simulink model "PID"  (R2024a)
settings: Solver=VariableStepAuto  StartTime=0.0  StopTime=11  RelTol=1e-3
settings Model: Creator=thunguyen  LastModifiedBy=thunguyen

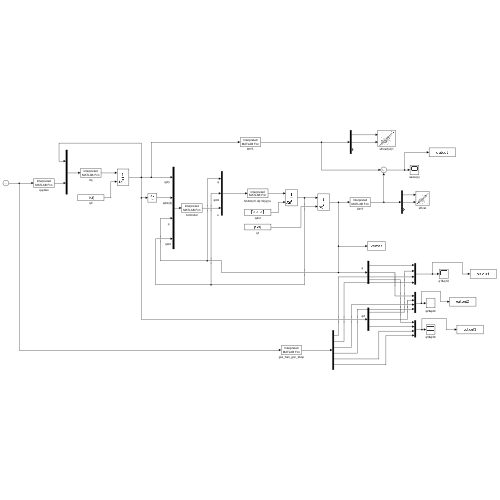
[thumbnail: Simulink's stored preview of the top-level diagram]
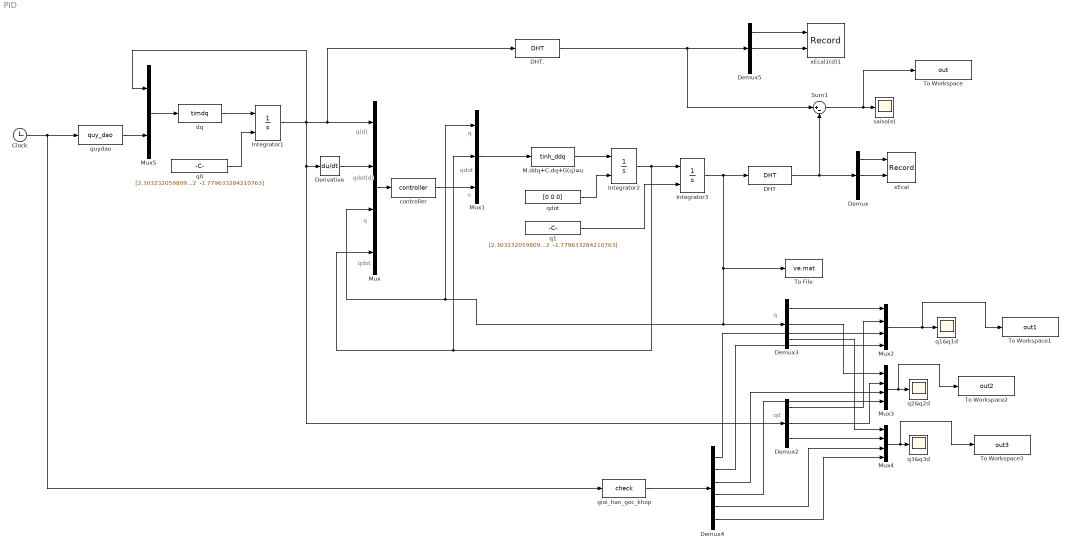
== system PID ==
  note: qd
  note: q
  note: u
  note: qdot
  note: qdot(d)
  note: q
  note: q
  note: q(d)
  note: qdot
  Clock : Clock
      settings: Decimation=2
  DHT : MATLABFcn  MATLABFcn=DHT  OutputDimensions=3  Output1D=off
  DHT. : MATLABFcn  MATLABFcn=DHT  OutputDimensions=3  Output1D=off
  Demux{,2..3,5} (4 alike) : Demux  Outputs=3
  Demux4 : Demux  Outputs=6
  Derivative : Derivative
  Integrator1 : Integrator  InitialConditionSource=external  InitialCondition=1
  Integrator2 : Integrator  InitialConditionSource=external  InitialCondition=1
  Integrator3 : Integrator  InitialConditionSource=external  InitialCondition=1
  M.ddq+C.dq+G(q)=u : MATLABFcn  MATLABFcn=tinh_ddq  OutputDimensions=3  Output1D=off
  Mux{,2..4} (4 alike) : Mux
  Mux1 : Mux  Inputs=3
  Mux5 : Mux  Inputs=2
  Sum1 : Sum  Inputs=|+-
  To File : ToFile  Filename=ve.mat
  To Workspace : ToWorkspace  VariableName=out  SaveFormat=Timeseries  SampleTime=-1
  To Workspace1 : ToWorkspace  VariableName=out1  SaveFormat=Timeseries  SampleTime=-1
  To Workspace2 : ToWorkspace  VariableName=out2  SaveFormat=Timeseries  SampleTime=-1
  To Workspace3 : ToWorkspace  VariableName=out3  SaveFormat=Timeseries  SampleTime=-1
  controller : MATLABFcn  MATLABFcn=controller  OutputDimensions=3  Output1D=off
  dq : MATLABFcn  MATLABFcn=timdq  OutputDimensions=3  Output1D=off
  gioi_han_goc_khop : MATLABFcn  MATLABFcn=check  OutputDimensions=6
  q0 : Constant  Value="[2.303232059809062   0.120492197697522  -1.779633284210763]"  VectorParams1D=off
  q1 : Constant  Value="[2.303232059809062   0.120492197697522  -1.779633284210763]"  VectorParams1D=off
  q1&q1d : Scope
  q2&q2d : Scope
  q3&q3d : Scope
  qdot : Constant  Value=[0 0 0]  VectorParams1D=off
  quydao : MATLABFcn  MATLABFcn=quy_dao  OutputDimensions=6
  saiso(e) : Scope
  xEcal : Record  FileSettingsInternal="{\"entries\":[{\"content\":{\"excelSettings\":{\"content\":{},\"type\":\"Streamout.ExcelSettings\"}},\"type\":\"Streamout.FileSettingStorage\",\"uuid\":\"\"}],\"packageUris\":[\"http:\\/\\/schema.mathworks.com\\/mf0\\/streamout_blocks\\/R2020a\"],\"version\":\"1.0\"}"  Layout=[1 1]  SignalsInternal="{\"entries\":[{\"content\":{\"signals\":[{\"content\":{\"blockPath\":[],\"dimensions\":[1],\"domain\":\"\",\"lineColor\":\"#77ac30\",\"lineWidth\":2,\"plots\":[ 1 ],\"port\":1,\"sid\":[\"\"],\"signalID\":1,\"signalName\":\"Demux:1\"},\"type\":\"RecordBlkView.Signal\",\"uuid\":\"\"},{\"content\":{\"blockPath\":[],\"dimensions\":[1],\"domain\":\"\",\"lineColor\":\"#4dbeee\",\"lineWidth\":2,\"plots\":[ 1 ],\"port\":2,\"sid\":[\"\"],\"signalID\":2,\"signalName\":\"Demux:2\"},\"type\":\"RecordBlkView.Signal\",\"uuid\":\"\"}]},\"type\":\"RecordBlkView.InputSignals\",\"uuid\":\"\"}],\"packageUris\":[\"http:\\/\\/schema.mathworks.com\\/mf0\\/streamout_blocks\\/R2020a\"],\"version\":\"1.0\"}"  VisualizationBindings="{\"xyplotplugin\":{\"info\":[{\"series\":[{\"bindingParametersList\":[{\"parameter\":\"X-Axis\",\"signalID\":1,\"signalName\":\"Demux:1\"},{\"parameter\":\"Y-Axis\",\"signalID\":2,\"signalName\":\"Demux:2\"}],\"seriesID\":0}],\"subplotID\":1}]}}"  CompatibilityTag=XY
  xEcal1(d)1 : Record  FileSettingsInternal="{\"entries\":[{\"content\":{\"excelSettings\":{\"content\":{},\"type\":\"Streamout.ExcelSettings\"}},\"type\":\"Streamout.FileSettingStorage\",\"uuid\":\"\"}],\"packageUris\":[\"http:\\/\\/schema.mathworks.com\\/mf0\\/streamout_blocks\\/R2020a\"],\"version\":\"1.0\"}"  Layout=[1 1]  SignalsInternal="{\"entries\":[{\"content\":{\"signals\":[{\"content\":{\"blockPath\":[],\"dimensions\":[1],\"domain\":\"\",\"lineColor\":\"#a2142f\",\"lineWidth\":2,\"plots\":[ 1 ],\"port\":1,\"sid\":[\"\"],\"signalID\":1,\"signalName\":\"Demux5:1\"},\"type\":\"RecordBlkView.Signal\",\"uuid\":\"\"},{\"content\":{\"blockPath\":[],\"dimensions\":[1],\"domain\":\"\",\"lineColor\":\"#139fff\",\"lineWidth\":2,\"plots\":[ 1 ],\"port\":2,\"sid\":[\"\"],\"signalID\":2,\"signalName\":\"Demux5:2\"},\"type\":\"RecordBlkView.Signal\",\"uuid\":\"\"}]},\"type\":\"RecordBlkView.InputSignals\",\"uuid\":\"\"}],\"packageUris\":[\"http:\\/\\/schema.mathworks.com\\/mf0\\/streamout_blocks\\/R2020a\"],\"version\":\"1.0\"}"  VisualizationBindings="{\"xyplotplugin\":{\"info\":[{\"series\":[{\"bindingParametersList\":[{\"parameter\":\"X-Axis\",\"signalID\":1,\"signalName\":\"Demux5:1\"},{\"parameter\":\"Y-Axis\",\"signalID\":2,\"signalName\":\"Demux5:2\"}],\"seriesID\":0}],\"subplotID\":1}]}}"  CompatibilityTag=XY
  wires:
  Clock/1 -> quydao/1, gioi_han_goc_khop/1
  DHT/1 -> Sum1/2, Demux/1
  Demux/1 -> xEcal/1
  Demux/2 -> xEcal/2
  M.ddq+C.dq+G(q)=u/1 -> Integrator2/1
  Integrator2/1 -> Integrator3/1, Mux1/2, Mux/4
  qdot/1 -> Integrator2/2
  Sum1/1 -> To Workspace/1, saiso(e)/1
  Mux/1 -> controller/1
  Mux1/1 -> M.ddq+C.dq+G(q)=u/1
  controller/1 -> Mux1/3
  Integrator3/1 -> DHT/1, To File/1, Mux/3, Mux1/1, Demux3/1
  Mux2/1 -> To Workspace1/1, q1&q1d/1
  Mux4/1 -> To Workspace3/1, q3&q3d/1
  Demux3/1 -> Mux2/1
  Demux2/1 -> Mux2/2
  Demux3/2 -> Mux3/1
  Demux2/2 -> Mux3/2
  Demux3/3 -> Mux4/1
  Demux2/3 -> Mux4/2
  Derivative/1 -> Mux/2
  Mux5/1 -> dq/1
  dq/1 -> Integrator1/1
  Integrator1/1 -> Mux5/1, Demux2/1, Derivative/1, DHT./1, Mux/1
  gioi_han_goc_khop/1 -> Demux4/1
  Demux4/1 -> Mux2/3
  Demux4/2 -> Mux2/4
  Demux4/3 -> Mux3/3
  Demux4/4 -> Mux3/4
  Demux4/5 -> Mux4/3
  Demux4/6 -> Mux4/4
  q1/1 -> Integrator3/2
  q0/1 -> Integrator1/2
  Demux5/1 -> xEcal1(d)1/1
  Demux5/2 -> xEcal1(d)1/2
  DHT./1 -> Sum1/1, Demux5/1
  quydao/1 -> Mux5/2
  Mux3/1 -> To Workspace2/1, q2&q2d/1
